simulink model "Wallnode_9node"  (R2018b)
settings: Solver=FixedStepAuto  StartTime=0.0  StopTime=100000  FixedStep=5  RelTol=1e-3
values from neighbouring files (symbols this model uses):
  wallU = 2.1    [PartitionWallMatrix.m]
undefined symbols (not defined in the file or in its folder): DiffuseHorizontal, DiscIntNeverNeededParam, DNI, NESW_wallArea, offsetDays, TemperatureSeries, Wall_Irradiance_Angles_NEWS, wallHeatCapacityExt, wallHeatCapacityInt, wallHeatCapacityMid, wallStartTempExt, windSpeedSeries
settings Model: Creator=cpp14rcj  LastModifiedBy=cpp14rcj

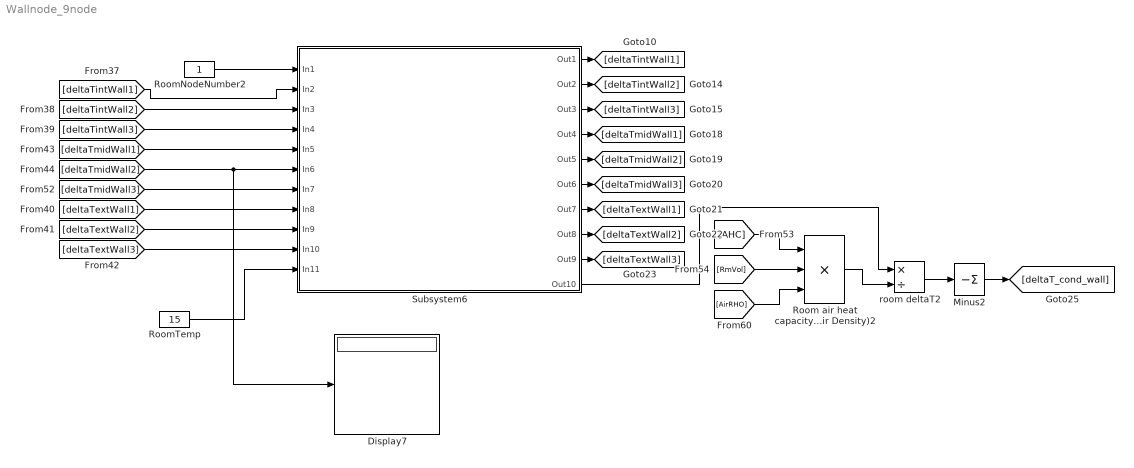
== system Wallnode_9node ==
  Display7 : Display
  Minus2 : Sum  Inputs=-
  Room air heat capacity (Cp*volume air*air Density)2 : Product  Inputs=***
  RoomNodeNumber2 : Constant
  RoomTemp : Constant  Value=15
  Subsystem6 : Subsystem
      mask Display:
      | disp('Wall Node \n Sub-Model')
      | port_label('input', 1, 'Room Node #')
      | port_label('input', 2, 'dT Internal 1 NEWS in')
      | port_label('input', 3, 'dT Internal 2 NEWS in')
      | port_label('input', 4, 'dT Internal 3 NEWS in')
      | port_label('input', 5, 'dT Mid 1 NEWS in')
      | port_label('input', 6, 'dT Mid 2 NEWS in')
      | port_label('input', 7, 'dT Mid 3 NEWS in')
      | port_label('input', 8, 'dT External 1 NEWS in')
      | port_label('input', 9, 'dT External 2 NEWS in')
      | port_label('input', 10, 'dT External 3 NEWS in')
      | port_label('input', 11, 'T_Room')
      | 
      | port_label('output', 1, 'dT Internal1 NEWS out')
      | port_label('output', 2, 'dT Internal2 NEWS out')
      | port_label('output', 3, 'dT Internal3 NEWS out')
      | port_label('output', 4, 'dT Mid1 NEWS out')
      | port_label('output', 5, 'dT Mid2 NEWS out')
      | port_label('output', 6, 'dT Mid3 NEWS out')
      | port_label('output', 7, 'dT External1 NEWS out')
      | port_label('output', 8, 'dT External2 NEWS out')
      | port_label('output', 9, 'dT External3 NEWS out')
      | port_label('output', 10, 'Total Qloss Through Walls')
  room deltaT2 : Product  Inputs=*/
  wires:
  Subsystem6/10(Out10) -> room deltaT2/1
  Subsystem6/8(Out8) -> [deltaTextWall2]
  RoomTemp/1 -> Subsystem6/11(In11)
  [deltaTmidWall1] -> Subsystem6/5(In5)
  Subsystem6/5(Out5) -> [deltaTmidWall2]
  [deltaTmidWall2] -> Display7/1, Subsystem6/6(In6)
  Subsystem6/2(Out2) -> [deltaTintWall2]
  Subsystem6/4(Out4) -> [deltaTmidWall1]
  [deltaTextWall1] -> Subsystem6/8(In8)
  [deltaTmidWall3] -> Subsystem6/7(In7)
  [deltaTextWall3] -> Subsystem6/10(In10)
  [deltaTintWall2] -> Subsystem6/3(In3)
  Subsystem6/9(Out9) -> [deltaTextWall3]
  room deltaT2/1 -> Minus2/1
  [AirRHO] -> Room air heat capacity (Cp*volume air*air Density)2/3
  [AHC] -> Room air heat capacity (Cp*volume air*air Density)2/1
  RoomNodeNumber2/1 -> Subsystem6/1(In1)
  Subsystem6/3(Out3) -> [deltaTintWall3]
  Subsystem6/1(Out1) -> [deltaTintWall1]
  Subsystem6/7(Out7) -> [deltaTextWall1]
  Minus2/1 -> [deltaT_cond_wall]
  [RmVol] -> Room air heat capacity (Cp*volume air*air Density)2/2
  Subsystem6/6(Out6) -> [deltaTmidWall3]
  [deltaTextWall2] -> Subsystem6/9(In9)
  [deltaTintWall1] -> Subsystem6/2(In2)
  Room air heat capacity (Cp*volume air*air Density)2/1 -> room deltaT2/2
  [deltaTintWall3] -> Subsystem6/4(In4)

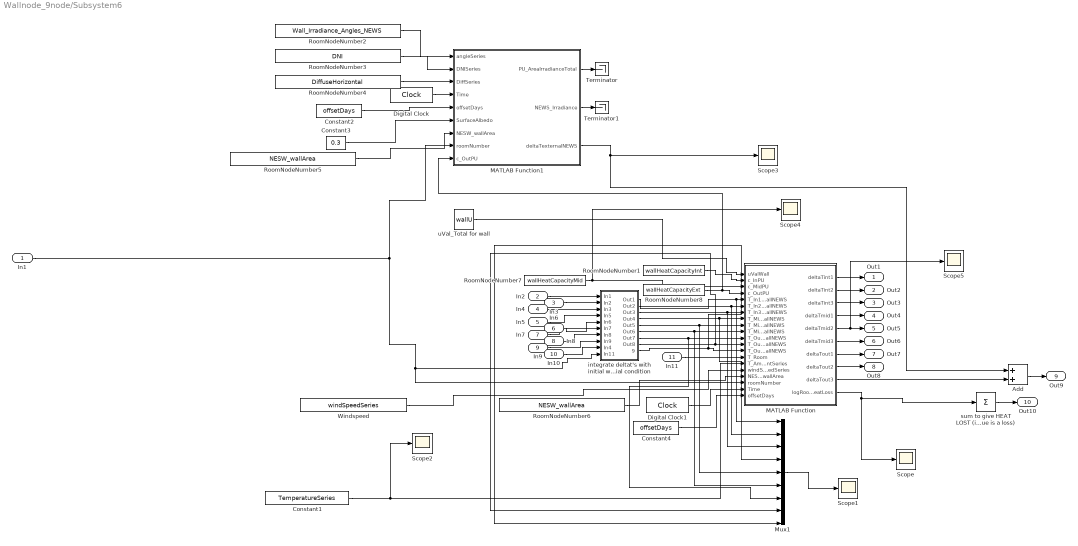
== system Wallnode_9node/Subsystem6 ==
  In1 : Inport
  In2 : Inport  Port=2
  In3 : Inport  Port=3
  In4 : Inport  Port=4
  In5 : Inport  Port=5
  In6 : Inport  Port=6
  In7 : Inport  Port=7
  In8 : Inport  Port=8
  In9 : Inport  Port=9
  In10 : Inport  Port=10
  In11 : Inport  Port=11
  Add : Sum
  Constant1 : Constant  Value=TemperatureSeries
  Constant2 : Constant  Value=offsetDays
  Constant3 : Constant  Value=0.3
  Constant4 : Constant  Value=offsetDays
  Digital Clock : DigitalClock  SampleTime=10
  Digital Clock1 : DigitalClock  SampleTime=10
  MATLAB Function : MATLAB Function  TreatAsAtomicUnit=on
  MATLAB Function1 : MATLAB Function  TreatAsAtomicUnit=on
  Mux1 : Mux  Inputs=9
  RoomNodeNumber1 : Constant  Value=wallHeatCapacityInt
  RoomNodeNumber2 : Constant  Value=Wall_Irradiance_Angles_NEWS
  RoomNodeNumber3 : Constant  Value=DNI
  RoomNodeNumber4 : Constant  Value=DiffuseHorizontal
  RoomNodeNumber5 : Constant  Value=NESW_wallArea
  RoomNodeNumber6 : Constant  Value=NESW_wallArea
  RoomNodeNumber7 : Constant  Value=wallHeatCapacityMid
  RoomNodeNumber8 : Constant  Value=wallHeatCapacityExt
  Scope{,1..5} (6 alike) : Scope
  Terminator : Terminator
  Terminator1 : Terminator
  Windspeed : Constant  Value=windSpeedSeries
  integrate deltat's with initial wall temps as initial condition : Subsystem
  sum to give HEAT LOST (i.e. positive value is a loss) : Sum  Inputs=+
  uVal_Total for wall : Constant  Value=wallU
  Out1 : Outport
  Out2 : Outport  Port=2
  Out3 : Outport  Port=3
  Out4 : Outport  Port=4
  Out5 : Outport  Port=5
  Out6 : Outport  Port=6
  Out7 : Outport  Port=7
  Out8 : Outport  Port=8
  Out9 : Outport  Port=9
  Out10 : Outport  Port=10
  wires:
  Constant1/1 -> Scope2/1, MATLAB Function/15(T_AmbientSeries)
  integrate deltat's with initial wall temps as initial condition/1(Out1) -> Mux1/1, MATLAB Function/5(T_In1WallNEWS)
  RoomNodeNumber2/1 -> MATLAB Function1/1(angleSeries)
  RoomNodeNumber1/1 -> MATLAB Function/2(c_InPU)
  MATLAB Function/3(deltaTint3) -> Out3/1
  In11/1 -> MATLAB Function/14(T_Room)
  MATLAB Function1/2(NEWS_Irradiance) -> Terminator1/1
  MATLAB Function/10(logRoomHeatLoss) -> sum to give HEAT LOST (i.e. positive value is a loss)/1, Scope/1
  RoomNodeNumber8/1 -> MATLAB Function/4(c_OutPU), MATLAB Function1/9(c_OutPU)
  uVal_Total for wall/1 -> MATLAB Function/1(uValWall)
  In4/1 -> integrate deltat's with initial wall temps as initial condition/3(In3)
  Digital Clock/1 -> MATLAB Function1/4(Time)
  integrate deltat's with initial wall temps as initial condition/2(Out2) -> Mux1/2, MATLAB Function/6(T_In2WallNEWS)
  RoomNodeNumber3/1 -> MATLAB Function1/2(DNISeries)
  integrate deltat's with initial wall temps as initial condition/3(Out3) -> Mux1/3, MATLAB Function/7(T_In3WallNEWS)
  MATLAB Function/1(deltaTint1) -> Out1/1
  MATLAB Function/9(deltaTout3) -> Add/2
  In3/1 -> integrate deltat's with initial wall temps as initial condition/2(In2)
  Windspeed/1 -> MATLAB Function/16(windSpeedSeries)
  Constant3/1 -> MATLAB Function1/6(SurfaceAlbedo)
  RoomNodeNumber4/1 -> MATLAB Function1/3(DiffSeries)
  In1/1 -> integrate deltat's with initial wall temps as initial condition/10(In11), MATLAB Function/18(roomNumber), MATLAB Function1/8(roomNumber)
  MATLAB Function1/3(deltaTexternalNEWS) -> Scope3/1, Add/1
  RoomNodeNumber5/1 -> MATLAB Function1/7(NESW_wallArea)
  RoomNodeNumber6/1 -> MATLAB Function/17(NESW_wallArea)
  Constant4/1 -> MATLAB Function/20(offsetDays)
  Constant2/1 -> MATLAB Function1/5(offsetDays)
  Digital Clock1/1 -> MATLAB Function/19(Time)
  MATLAB Function1/1(PU_AreaIrradianceTotal) -> Terminator/1
  In2/1 -> integrate deltat's with initial wall temps as initial condition/1(In1)
  MATLAB Function/2(deltaTint2) -> Out2/1
  sum to give HEAT LOST (i.e. positive value is a loss)/1 -> Out10/1
  MATLAB Function/4(deltaTmid1) -> Out4/1
  MATLAB Function/5(deltaTmid2) -> Scope5/1, Out5/1
  MATLAB Function/6(deltaTmid3) -> Out6/1
  MATLAB Function/7(deltaTout1) -> Out7/1
  MATLAB Function/8(deltaTout2) -> Out8/1
  Add/1 -> Out9/1
  In5/1 -> integrate deltat's with initial wall temps as initial condition/4(In5)
  In6/1 -> integrate deltat's with initial wall temps as initial condition/5(In6)
  In7/1 -> integrate deltat's with initial wall temps as initial condition/6(In7)
  In8/1 -> integrate deltat's with initial wall temps as initial condition/7(In8)
  In9/1 -> integrate deltat's with initial wall temps as initial condition/8(In9)
  In10/1 -> integrate deltat's with initial wall temps as initial condition/9(In4)
  integrate deltat's with initial wall temps as initial condition/4(Out4) -> MATLAB Function/8(T_Mid1WallNEWS), Mux1/4
  integrate deltat's with initial wall temps as initial condition/5(Out5) -> MATLAB Function/9(T_Mid2WallNEWS), Mux1/5
  integrate deltat's with initial wall temps as initial condition/6(Out6) -> MATLAB Function/10(T_Mid3WallNEWS), Mux1/6
  integrate deltat's with initial wall temps as initial condition/7(Out7) -> MATLAB Function/11(T_Out1WallNEWS), Mux1/7
  integrate deltat's with initial wall temps as initial condition/8(Out8) -> Mux1/8, MATLAB Function/12(T_Out2WallNEWS)
  integrate deltat's with initial wall temps as initial condition/9(Out10) -> Mux1/9, MATLAB Function/13(T_Out3WallNEWS)
  Mux1/1 -> Scope1/1
  RoomNodeNumber7/1 -> Scope4/1, MATLAB Function/3(c_MidPU)

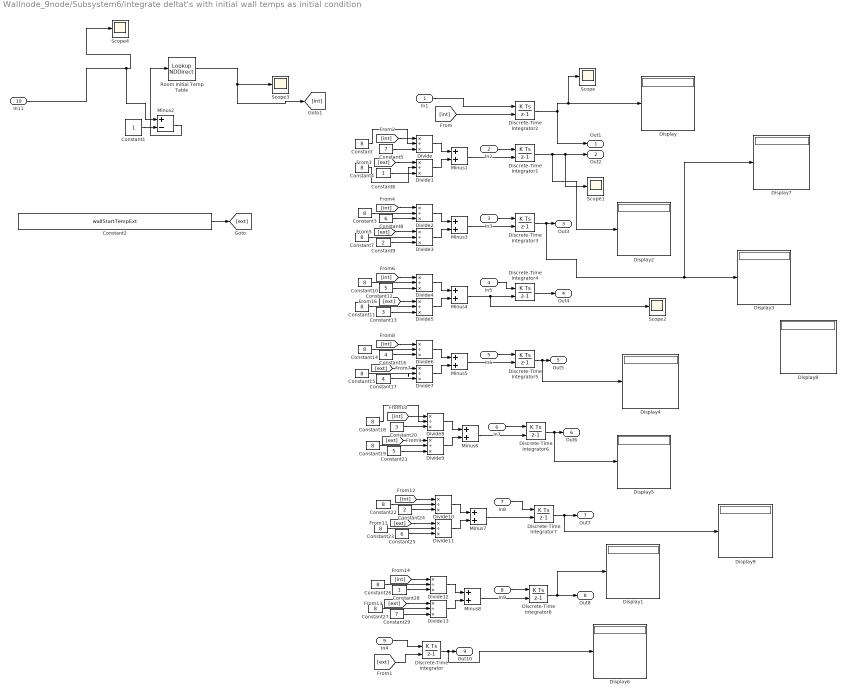
== system Wallnode_9node/Subsystem6/integrate deltat's with initial wall temps as initial condition ==
  In1 : Inport
  In2 : Inport  Port=2
  In3 : Inport  Port=3
  In5 : Inport  Port=4
  In6 : Inport  Port=5
  In7 : Inport  Port=6
  In8 : Inport  Port=7
  In9 : Inport  Port=8
  In4 : Inport  Port=9
  In11 : Inport  Port=10
  Constant{,3..4,7,10..11,14..15,18..19,22..23,26..27} (14 alike) : Constant  Value=8
  Constant1 : Constant
  Constant12 : Constant  Value=5
  Constant13 : Constant  Value=3
  Constant16 : Constant  Value=4
  Constant17 : Constant  Value=4
  Constant2 : Constant  Value=wallStartTempExt
  Constant20 : Constant  Value=3
  Constant21 : Constant  Value=5
  Constant24 : Constant  Value=2
  Constant25 : Constant  Value=6
  Constant28 : Constant
  Constant29 : Constant  Value=7
  Constant5 : Constant  Value=7
  Constant6 : Constant
  Constant8 : Constant  Value=6
  Constant9 : Constant  Value=2
  Discrete-Time Integrator{,1..8} (9 alike) : DiscreteIntegrator  InitialConditionSource=external  SampleTime=-1  ICPrevOutput=DiscIntNeverNeededParam  ICPrevScaledInput=DiscIntNeverNeededParam
  Display{,1..9} (10 alike) : Display
  Divide{,1..13} (14 alike) : Product  Inputs=*/*
  Minus{1,3..8} (7 alike) : Sum
  Minus2 : Sum  Inputs=+-
  Room Initial Temp Table : LookupNDDirect  NumberOfTableDimensions=1  Table=wallStartTempInt'
  Scope{,1..4} (5 alike) : Scope
  Out1 : Outport
  Out2 : Outport  Port=2
  Out3 : Outport  Port=3
  Out4 : Outport  Port=4
  Out5 : Outport  Port=5
  Out6 : Outport  Port=6
  Out7 : Outport  Port=7
  Out8 : Outport  Port=8
  Out10 : Outport  Port=9
  wires:
  Discrete-Time Integrator1/1 -> Display2/1, Scope1/1, Out2/1
  Discrete-Time Integrator2/1 -> Out1/1, Scope/1, Display/1
  Room Initial Temp Table/1 -> [int], Scope3/1
  In2/1 -> Discrete-Time Integrator1/1
  Constant2/1 -> [ext]
  In1/1 -> Discrete-Time Integrator2/1
  In11/1 -> Scope4/1, Minus2/1
  Constant1/1 -> Minus2/2
  Minus2/1 -> Room Initial Temp Table/1
  [int] -> Discrete-Time Integrator2/2
  [ext] -> Discrete-Time Integrator/2
  Divide/1 -> Minus1/1
  Divide1/1 -> Minus1/2
  Constant/1 -> Divide/2
  Constant4/1 -> Divide1/2
  [int] -> Divide/1
  [ext] -> Divide1/1
  Constant5/1 -> Divide/3
  Constant6/1 -> Divide1/3
  Minus1/1 -> Discrete-Time Integrator1/2
  Minus3/1 -> Discrete-Time Integrator3/2
  Constant9/1 -> Divide3/3
  [ext] -> Divide3/1
  Constant8/1 -> Divide2/3
  [int] -> Divide2/1
  Constant7/1 -> Divide3/2
  Constant3/1 -> Divide2/2
  Divide3/1 -> Minus3/2
  Divide2/1 -> Minus3/1
  Minus4/1 -> Scope2/1, Discrete-Time Integrator4/2
  Constant13/1 -> Divide5/3
  [ext] -> Divide5/1
  Constant12/1 -> Divide4/3
  [int] -> Divide4/1
  Constant11/1 -> Divide5/2
  Constant10/1 -> Divide4/2
  Divide5/1 -> Minus4/2
  Divide4/1 -> Minus4/1
  Minus5/1 -> Discrete-Time Integrator5/2
  Constant17/1 -> Divide7/3
  [ext] -> Divide7/1
  Constant16/1 -> Divide6/3
  [int] -> Divide6/1
  Constant15/1 -> Divide7/2
  Constant14/1 -> Divide6/2
  Divide7/1 -> Minus5/2
  Divide6/1 -> Minus5/1
  In3/1 -> Discrete-Time Integrator3/1
  In5/1 -> Discrete-Time Integrator4/1
  In6/1 -> Discrete-Time Integrator5/1
  Divide8/1 -> Minus6/1
  Constant19/1 -> Divide9/2
  Constant18/1 -> Divide8/2
  Divide9/1 -> Minus6/2
  [ext] -> Divide9/1
  Constant21/1 -> Divide9/3
  Minus6/1 -> Discrete-Time Integrator6/2
  Constant20/1 -> Divide8/3
  [int] -> Divide8/1
  Divide10/1 -> Minus7/1
  Constant23/1 -> Divide11/2
  Constant22/1 -> Divide10/2
  Divide11/1 -> Minus7/2
  [ext] -> Divide11/1
  Constant25/1 -> Divide11/3
  Minus7/1 -> Discrete-Time Integrator7/2
  Constant24/1 -> Divide10/3
  [int] -> Divide10/1
  Divide12/1 -> Minus8/1
  Constant27/1 -> Divide13/2
  Constant26/1 -> Divide12/2
  Divide13/1 -> Minus8/2
  [ext] -> Divide13/1
  Constant29/1 -> Divide13/3
  Minus8/1 -> Discrete-Time Integrator8/2
  Constant28/1 -> Divide12/3
  [int] -> Divide12/1
  In7/1 -> Discrete-Time Integrator6/1
  In8/1 -> Discrete-Time Integrator7/1
  In9/1 -> Discrete-Time Integrator8/1
  Discrete-Time Integrator3/1 -> Display7/1, Display3/1, Out3/1
  Discrete-Time Integrator4/1 -> Out4/1
  Discrete-Time Integrator6/1 -> Display5/1, Out6/1
  Discrete-Time Integrator7/1 -> Display9/1, Out7/1
  Discrete-Time Integrator8/1 -> Display1/1, Out8/1
  Discrete-Time Integrator/1 -> Display6/1, Out10/1
  In4/1 -> Discrete-Time Integrator/1
  Discrete-Time Integrator5/1 -> Display4/1, Out5/1

== matlab function Wallnode_9node/Subsystem6/MATLAB Function ==
  data: uValWall input; deltaTint1 output; deltaTint2 output; deltaTint3 output; c_InPU input; c_MidPU input; c_OutPU input; T_In1WallNEWS input; T_In2WallNEWS input; T_In3WallNEWS input; T_Mid1WallNEWS input; T_Mid2WallNEWS input; T_Mid3WallNEWS input; T_Out1WallNEWS input; T_Out2WallNEWS input; T_Out3WallNEWS input; T_Room input; T_AmbientSeries input; windSpeedSeries input; deltaTmid1 output; deltaTmid2 output; deltaTmid3 output; deltaTout1 output; deltaTout2 output; deltaTout3 output; NESW_wallArea input; roomNumber input; logRoomHeatLoss output; Time input; offsetDays input
function [deltaTint1,deltaTint2,deltaTint3,deltaTmid1,deltaTmid2,deltaTmid3,deltaTout1,deltaTout2,deltaTout3,logRoomHeatLoss] = fcn(uValWall,c_InPU,c_MidPU,c_OutPU,T_In1WallNEWS,T_In2WallNEWS,T_In3WallNEWS, T_Mid1WallNEWS,T_Mid2WallNEWS,T_Mid3WallNEWS,T_Out1WallNEWS,T_Out2WallNEWS,T_Out3WallNEWS,T_Room,T_AmbientSeries,windSpeedSeries,NESW_wallArea,roomNumber,Time,offsetDays)




  deltaTint1=zeros(1,4);
  deltaTint2=zeros(1,4);
  deltaTint3=zeros(1,4);
   deltaTmid1=zeros(1,4);
   deltaTmid2=zeros(1,4);
   deltaTmid3=zeros(1,4);
    deltaTout1=zeros(1,4);
    deltaTout2=zeros(1,4);
    deltaTout3=zeros(1,4);
    logRoomHeatLoss=zeros(1,4);

    v_Wind=windSpeedSeries(ceil((offsetDays*1440)+Time/60+0.00001),1);
   T_Ambient=T_AmbientSeries(ceil((offsetDays*1440)+Time/60+0.00001),1);
    
k=uValWall*8;



NEWS_wallArea=NESW_wallArea;
NEWS_wallArea([3 4],:)=NEWS_wallArea([4 3],:);
RoomWallAreas_NEWS=NEWS_wallArea(:,roomNumber)';


for i=1:4
    
    if RoomWallAreas_NEWS(1,i)>0

c_In=c_InPU*RoomWallAreas_NEWS(1,i);
c_Mid=c_MidPU*RoomWallAreas_NEWS(1,i);
c_Out=c_OutPU*RoomWallAreas_NEWS(1,i);




T_In1Wall=T_In1WallNEWS(1,i);
T_In2Wall=T_In2WallNEWS(1,i);
T_In3Wall=T_In3WallNEWS(1,i);
T_Mid1Wall=T_Mid1WallNEWS(1,i);
T_Mid2Wall=T_Mid2WallNEWS(1,i);
T_Mid3Wall=T_Mid3WallNEWS(1,i);
T_Out1Wall=T_Out1WallNEWS(1,i);
T_Out2Wall=T_Out2WallNEWS(1,i);
T_Out3Wall=T_Out3WallNEWS(1,i);

aA=[-(k*RoomWallAreas_NEWS(1,i))/(c_In/3) (k*RoomWallAreas_NEWS(1,i))/(c_In/3)   0                                     0                                       0                                       0                                       0                                       0                                       0
   (k*RoomWallAreas_NEWS(1,i))/(c_In/3)   -(2*k*RoomWallAreas_NEWS(1,i))/(c_In/3)  (k*RoomWallAreas_NEWS(1,i))/(c_In/3)  0                                       0                                       0                                       0                                       0                                       0
   0                                      (k*RoomWallAreas_NEWS(1,i))/(c_In/3)   -(2*k*RoomWallAreas_NEWS(1,i))/(c_In/3) (k*RoomWallAreas_NEWS(1,i))/(c_In/3)    0                                       0                                       0                                       0                                       0
   0                                      0                                      (k*RoomWallAreas_NEWS(1,i))/(c_Mid/3) -(2*k*RoomWallAreas_NEWS(1,i))/(c_Mid/3)  (k*RoomWallAreas_NEWS(1,i))/(c_Mid/3)   0                                       0                                       0                                       0
   0                                      0                                      0                                     (k*RoomWallAreas_NEWS(1,i))/(c_Mid/3)   -(2*k*RoomWallAreas_NEWS(1,i))/(c_Mid/3)  (k*RoomWallAreas_NEWS(1,i))/(c_Mid/3)   0                                       0                                       0
   0                                      0                                      0                                     0                                       (k*RoomWallAreas_NEWS(1,i))/(c_Mid/3)   -(2*k*RoomWallAreas_NEWS(1,i))/(c_Mid/3)  (k*RoomWallAreas_NEWS(1,i))/(c_Mid/3)   0                                       0
   0                                      0                                      0                                     0                                       0                                       (k*RoomWallAreas_NEWS(1,i))/(c_Out/3)   -(2*k*RoomWallAreas_NEWS(1,i))/(c_Out/3)  (k*RoomWallAreas_NEWS(1,i))/(c_Out/3)   0       
   0                                      0                                      0                                     0                                       0                                       0                                       (k*RoomWallAreas_NEWS(1,i))/(c_Out/3)   -(2*k*RoomWallAreas_NEWS(1,i))/(c_Out/3)  (k*RoomWallAreas_NEWS(1,i))/(c_Out/3)                    
   0                                      0                                      0                                     0                                       0                                       0                                       0                                       (k*RoomWallAreas_NEWS(1,i))/(c_Out/3)   -(k*RoomWallAreas_NEWS(1,i))/(c_Out/3)]; 

bA=[1/(c_In/3) 0           0                0            0              0              0              0            0
    0          1/(c_In/3)  0                0            0              0              0              0            0
    0          0           1/(c_In/3)       0            0              0              0              0            0
    0          0           0                1/(c_Mid/3)  0              0              0              0            0
    0          0           0                0            1/(c_Mid/3)    0              0              0            0
    0          0           0                0            0              1/(c_Mid/3)    0              0            0
    0          0           0                0            0              0              1/(c_Out/3)    0            0
    0          0           0                0            0              0              0              1/(c_Out/3)  0          
    0          0           0                0            0              0              0              0            1/(c_Out/3)];
    
ab=[T_In1Wall
T_In2Wall
T_In3Wall
T_Mid1Wall
T_Mid2Wall
T_Mid3Wall
T_Out1Wall
T_Out2Wall
T_Out3Wall];

bb=[(2.5*(T_Room-T_In1Wall)+5.6*(T_Room-T_In1Wall))*RoomWallAreas_NEWS(1,i)
0 
0
0
0
0
0
0
(2.8+3*v_Wind)*(T_Ambient-T_Out3Wall)+5.6*(T_Ambient-T_Out3Wall)*RoomWallAreas_NEWS(1,i)];

test=bA*bb;
deltaT=aA*ab+bA*bb;

        deltaTint1(1,i)=deltaT(1,1);
        deltaTint2(1,i)=deltaT(2,1);
        deltaTint3(1,i)=deltaT(3,1);
        deltaTmid1(1,i)=deltaT(4,1);
        deltaTmid2(1,i)=deltaT(5,1);
        deltaTmid3(1,i)=deltaT(6,1);
        deltaTout1(1,i)=deltaT(7,1);
        deltaTout2(1,i)=deltaT(8,1);
        deltaTout3(1,i)=deltaT(9,1);
    
    logRoomHeatLoss(1,i)=bb(1,1);
    
    else
        
        
        
    logRoomHeatLoss(1,i)=0;
    
    end
    
end

== matlab function Wallnode_9node/Subsystem6/MATLAB Function1 ==
  data: PU_AreaIrradianceTotal output; angleSeries input; NEWS_Irradiance output; DNISeries input; DiffSeries input; Time input; offsetDays input; SurfaceAlbedo input; NESW_wallArea input; roomNumber input; c_OutPU input; deltaTexternalNEWS output
function [PU_AreaIrradianceTotal, NEWS_Irradiance,deltaTexternalNEWS] = SolarSeriesToExtWallGains(angleSeries,DNISeries,DiffSeries,Time,offsetDays,SurfaceAlbedo,NESW_wallArea,roomNumber,c_OutPU)

%deltaTexternalNEWS=zeros(1,4);

Angle_NEWS=angleSeries(ceil((offsetDays*1440)+Time/60+0.00001),1:4);
DNI=DNISeries(ceil((offsetDays*1440)+Time/60+0.00001),1);

PU_AreaDiff=DiffSeries(ceil((offsetDays*1440)+Time/60+0.00001),1)/2;%extracts correct Diff for the timestep, factor of 1/2 corrects for 90 degree walls (so only half Diff irradiance can be utilised)
PU_AreaDNI=cos(deg2rad(Angle_NEWS))*DNI;
NEWS_wallArea=NESW_wallArea;
NEWS_wallArea([3 4],:)=NEWS_wallArea([4 3],:);

RoomWallAreas_NEWS=NEWS_wallArea(:,roomNumber)';
PU_AreaIrradianceTotal=(PU_AreaDNI+PU_AreaDiff)*(1-SurfaceAlbedo);

NEWS_Irradiance=RoomWallAreas_NEWS.*PU_AreaIrradianceTotal;
deltaTexternalNEWS=NEWS_Irradiance./(c_OutPU*RoomWallAreas_NEWS);

for i=1:4
   
    if RoomWallAreas_NEWS(1,i)==0
        deltaTexternalNEWS(1,i)=0;
    else
        
    end
    
end
